simulink model "piLidar"  (R2022b)
settings: Solver=FixedStepAuto  StartTime=0.0  StopTime=inf  FixedStep=0.01  RelTol=1e-3  EnableMultiTasking=on
InitFcn:
  | Ts = 0.01;
model workspace (MAT data in the model file):
  SL_ROS_VariableLengthArrays_MaxSizes.CommonInfo.ArrayTruncateAction = 'EmitWarning'
  SL_ROS_VariableLengthArrays_MaxSizes.MsgTypeMap = containers.Map
  SL_ROS_VariableLengthArrays_MaxSizes.MsgTypeMap.serialization.keys = {'sensor_msgs/LaserScan', 'std_msgs/Header'}
  SL_ROS_VariableLengthArrays_MaxSizes.MsgTypeMap.serialization.values{1}(1).PropertyName = 'Intensities'
  SL_ROS_VariableLengthArrays_MaxSizes.MsgTypeMap.serialization.values{1}(1).DataType = 'single'
  SL_ROS_VariableLengthArrays_MaxSizes.MsgTypeMap.serialization.values{1}(1).MaxLength = 40
  SL_ROS_VariableLengthArrays_MaxSizes.MsgTypeMap.serialization.values{1}(2).PropertyName = 'Ranges'
  SL_ROS_VariableLengthArrays_MaxSizes.MsgTypeMap.serialization.values{1}(2).DataType = 'single'
  SL_ROS_VariableLengthArrays_MaxSizes.MsgTypeMap.serialization.values{1}(2).MaxLength = 40
  SL_ROS_VariableLengthArrays_MaxSizes.MsgTypeMap.serialization.values{2}.PropertyName = 'FrameId'
  SL_ROS_VariableLengthArrays_MaxSizes.MsgTypeMap.serialization.values{2}.DataType = 'uint8'
  SL_ROS_VariableLengthArrays_MaxSizes.MsgTypeMap.serialization.values{2}.MaxLength = 11
  SL_ROS_VariableLengthArrays_MaxSizes.MsgTypeMap.serialization.uniformity = 0
  SL_ROS_VariableLengthArrays_MaxSizes.MsgTypeMap.serialization.keyType = 'char'
  SL_ROS_VariableLengthArrays_MaxSizes.MsgTypeMap.serialization.valueType = 'any'
libraries: raspberrypiCommlib x2
settings Model: Creator=System-10  LastModifiedBy=System-10
settings SolverCC: PositivePriorityOrder=on
settings OptimizationCC: EnhancedBackFolding=on  PassReuseOutputArgsAs=Individual arguments  ZeroExternalMemoryAtStartup=off  ZeroInternalMemoryAtStartup=off  MaxStackSize=64  OptimizeBlockOrder=speed  DifferentSizesBufferReuse=on  OptimizationCustomize=off  EfficientTunableParamExpr=on
settings DebuggingCC: ParameterTunabilityLossMsg=error
settings HardwareCC: ProdBitPerPointer=32  ProdBitPerSizeT=32  ProdBitPerPtrDiffT=32  ProdLargestAtomicInteger=Long  ProdLargestAtomicFloat=Double  ProdWordSize=32  ProdLongLongMode=on  ProdHWDeviceType=ARM Compatible->ARM Cortex
settings RTWCC: Description=Embedded Coder  SystemTargetFile=ert.tlc  HardwareBoard=Raspberry Pi  TLCOptions="-aInlineSetEventsForThisBaseRateFcn=TLC_FALSE -aSuppressMultiTaskScheduler=TLC_FALSE  -aRateBasedStepFcn=0"  TemplateMakefile=ert_default_tmf  Toolchain=GNU GCC Embedded Linux  BuildConfiguration=Faster Runs
settings CodeAppCC: ForceParamTrailComments=on  IgnoreCustomStorageClasses=off  OperatorAnnotations=on  SimulinkDataObjDesc=on  SFDataObjDesc=on  InsertBlockDesc=on
settings ERTTargetCC: SupportVariableSizeSignals=on  ExtModeTransport=2  ExtModeStaticAlloc=on  ExtModeMexFile=ext_xcp  ExtModeIntrfLevel=Level2 - Open

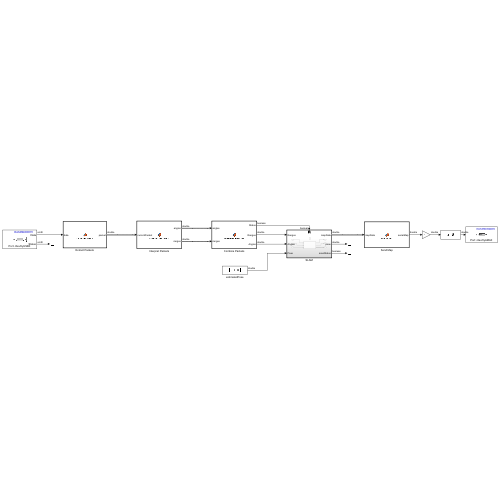
[thumbnail: Simulink's stored preview of the top-level diagram]
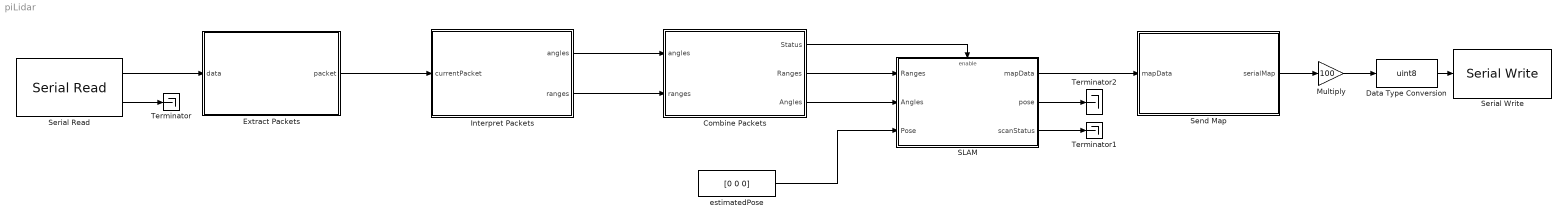
== system piLidar ==
  Combine Packets : MATLAB Function  TreatAsAtomicUnit=on
  Data Type Conversion : DataTypeConversion  OutDataTypeStr=uint8  SaturateOnIntegerOverflow=off  RndMeth=Floor
  Extract Packets : MATLAB Function  TreatAsAtomicUnit=on
  Interpret Packets : MATLAB Function  TreatAsAtomicUnit=on
  Multiply : Gain  Gain=100
  SLAM : Subsystem
  Send Map : MATLAB Function  TreatAsAtomicUnit=on
  Serial Read : raspberrypiCommlib/Serial Read  board=Pi 4 Model B  SCIModule_=/dev/ttyUSB0  Baudrate_=115200  Parity=None  StopBits_=1  HardwareFlowControl=None  ByteOrder=LittleEndian  DataLength=2000  DataType=uint8  OutputStatus=on  SampleTime=Ts  blockPlatform=RaspberryPi
  Serial Write : raspberrypiCommlib/Serial Write  board=Pi 4 Model B  SCIModule_=/dev/ttyAMA0  Baudrate_=115200  Parity=None  StopBits_=1  HardwareFlowControl=None  ByteOrder=LittleEndian  OutputStatus=off  blockPlatform=RaspberryPi
  Terminator : Terminator
  Terminator1 : Terminator
  Terminator2 : Terminator
  estimatedPose : Constant  Value=[0 0 0]
  wires:
  Serial Read/1 -> Extract Packets/1(data)
  estimatedPose/1 -> SLAM/3(Pose)
  Interpret Packets/2(ranges) -> Combine Packets/2(ranges)
  Combine Packets/2(Ranges) -> SLAM/1(Ranges)
  Interpret Packets/1(angles) -> Combine Packets/1(angles)
  Combine Packets/3(Angles) -> SLAM/2(Angles)
  Combine Packets/1(Status) -> SLAM/Enable
  Extract Packets/1(packet) -> Interpret Packets/1(currentPacket)
  Serial Read/2 -> Terminator/1
  SLAM/3(scanStatus) -> Terminator1/1
  SLAM/2(pose) -> Terminator2/1
  SLAM/1(mapData) -> Send Map/1(mapData)
  Send Map/1(serialMap) -> Multiply/1
  Multiply/1 -> Data Type Conversion/1
  Data Type Conversion/1 -> Serial Write/1

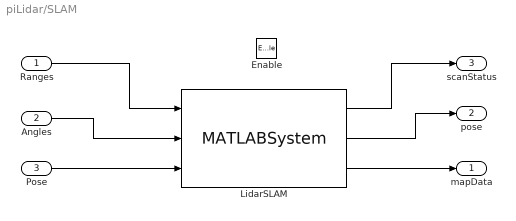
== system piLidar/SLAM ==
  Ranges : Inport
  Angles : Inport  Port=2
  Pose : Inport  Port=3
  Enable : EnablePort  PropagateVarSize=During execution
  LidarSLAM : MATLABSystem  System=LidarSlam_interp  SimulateUsing=Interpreted execution
      mask Type: LidarSlam_interp
      mask Display:
      | disp('LidarSlam_interp');
      | port_label('input',1,'ranges');
      | port_label('input',2,'angles');
      | port_label('input',3,'relPoseEst');
      | port_label('output',1,'isScanAdded');
      | port_label('output',2,'pose');
      | port_label('output',3,'mapData');
  mapData : Outport
  pose : Outport  Port=2
  scanStatus : Outport  Port=3
  wires:
  Ranges/1 -> LidarSLAM/1
  Angles/1 -> LidarSLAM/2
  LidarSLAM/2 -> pose/1
  LidarSLAM/1 -> scanStatus/1
  LidarSLAM/3 -> mapData/1
  Pose/1 -> LidarSLAM/3

== matlab function piLidar/Extract Packets ==
  settings: updateMethod=DISCRETE  sampleTime=Ts
  data: data input; packet output double size=[100 100]
function packet = extractPackets(data)
    
    persistent indicesOfHeaders;
    persistent startIdx;
    persistent endIdx;
    persistent idx;
    persistent zeroData;

    if isempty(zeroData)
        zeroData = uint8(zeros(1,size(data,2)));
    end

    data  = data';

    if isempty(indicesOfHeaders) || ~isequal(data, zeroData)
        
        indicesOfAA = find(data == 170);
        indicesOfHeaders = zeros(1, length(indicesOfAA)); 
        count = 0;
        
        startIdx = 0;
        endIdx = 0;
        idx = 0;

        for i = 1:length(indicesOfAA)
            if indicesOfAA(i) < length(data) && data(indicesOfAA(i) + 1) == 85
                count = count + 1;
                indicesOfHeaders(count) = indicesOfAA(i);
            end
        end

        indicesOfHeaders = indicesOfHeaders(1:count);   
    end
    
    if endIdx < indicesOfHeaders(end)
        idx = idx + 1;
        startIdx = indicesOfHeaders(idx);
        endIdx = indicesOfHeaders(idx+1);
        packet = double(data(startIdx:endIdx-1));
    else
        packet = [];
    end
end

== matlab function piLidar/Interpret Packets ==
  settings: updateMethod=DISCRETE  sampleTime=Ts
  data: currentPacket input; angles output size=[1 40]; ranges output size=[1 40]
function [angles, ranges] = interpretPackets(currentPacket)

    if size(currentPacket, 2) < 90
        angles = [];
        ranges = [];
        return;
    end

    FSA = double(bitor(bitshift(uint16(currentPacket(1, 6)), 8), uint16(currentPacket(1, 5)), 'uint16'));
    LSA = double(bitor(bitshift(uint16(currentPacket(1, 8)), 8), uint16(currentPacket(1, 7)), 'uint16'));
    
    AngleFSA = double(bitshift(FSA, -1) / 64);
    AngleLSA = double(bitshift(LSA, -1) / 64);
    diffAngle = mod((AngleLSA - AngleFSA),360);
    
    rawSi = uint8(currentPacket(:, 11:end));
    
    Si = zeros(1, 40);
    for i = 1:2:length(rawSi)
        Si((i + 1) / 2) = double(bitor(bitshift(uint16(rawSi(1, i + 1)), 8), uint16(rawSi(1, i)), 'uint16'));
    end
    
    AngleSi = zeros(1, 40);
    if Si(1) == 0
        AngleSi(1) = AngleFSA;
    else
        AngleSi(1) = AngleFSA + atan(21.8*((155.3-Si(1))/(155.3*Si(1))));
    end

    for i = 2:39
        if Si(i) == 0
            AngleSi(i) = ((diffAngle / (40 - 1)) * (i - 1) + AngleFSA);
        else
            AngleSi(i) = ((diffAngle / (40 - 1)) * (i - 1) + AngleFSA) + atan(21.8*((155.3-Si(i))/(155.3*Si(i))));
        end
    end

    if Si(40) == 0
        AngleSi(40) = AngleLSA;
    else
        AngleSi(40) = AngleLSA + atan(21.8*((155.3-Si(end))/(155.3*Si(end))));
    end

    %Current Angles as 1x40 array [deg].
    angles = AngleSi;

    %Current Ranges as 1x40 array [meter].
    Si = Si / 4000;
    ranges = Si;
end

== matlab function piLidar/Combine Packets ==
  settings: updateMethod=DISCRETE  sampleTime=Ts
  data: Status output boolean; Ranges output size=[1 400]; angles input; Angles output size=[1 400]; ranges input
function [Status,Ranges,Angles]  = combinePackets(angles,ranges)
    persistent count; 
    persistent elemAngles;
    persistent elemRanges;

    if isempty(count)
        count = 0;
        elemAngles = zeros(1,400);
        elemRanges = zeros(1,400);
    end
        
    for i = 1:length(angles)
        elemAngles(i+count) = angles(i);
        elemRanges(i+count) = ranges(i);
    end
    if count < (length(elemAngles)-length(angles))
        count = count + length(angles);
        Angles = zeros(1,400);
        Ranges = zeros(1,400);
        Status = boolean(0);
    else
        count = 0;
        %Current Angles as 1x400 array [rad].
        Angles = deg2rad(elemAngles);
        %Current Ranges as 1x400 array [meter].
        Ranges = elemRanges;
        Status = boolean(1);
    end
end

== matlab function piLidar/Send Map ==
  settings: updateMethod=DISCRETE  sampleTime=Ts
  data: mapData input; serialMap output double
function serialMap = sendMap(mapData)
    persistent currentColumn;
    persistent idxRow;
    persistent currentMap;

    if isempty(currentColumn)
        currentColumn = 0.5*ones(1,340);
        idxRow = 1;
        currentMap = mapData;
    end

    if ~(isequal(mapData, currentMap))
        currentMap = mapData;
        idxRow = 1;
    end

    for i = 1:size(currentMap,2)
        currentColumn(i) = currentMap(idxRow,i);
    end
    if idxRow <= size(mapData,1)
        idxRow = idxRow + 1;
        serialMap = (currentColumn);
    else
        serialMap = (0.5*ones(1,340));
    end
end
